simulink model "Nonlinear_PolePlacement"  (R2019b)
settings: Solver=VariableStepAuto  StartTime=0.0  StopTime=10.0  RelTol=1e-3
values from neighbouring files (symbols this model uses):
  b = 0.2    [HOMEWORK..m]
  g = 9.81    [HOMEWORK..m]
  Ktest = place(A,B,p)    [HOMEWORK..m]
  M = M_1*1.05+m    (= 11.3)    [HOMEWORK..m]
  m = 1.64    [HOMEWORK..m]
  Nu = NxNu(5)    [HOMEWORK..m]
  Nx = NxNu(1:4,:)    [HOMEWORK..m]
  x_0_1 = -0.01    [HOMEWORK..m]
  x_0_2 = 0.01    [HOMEWORK..m]
  x_0_3 = 0.05    [HOMEWORK..m]
  x_0_4 = 0.1    [HOMEWORK..m]
undefined symbols (not defined in the file or in its folder): J, L
settings Model: Creator=Sina  LastModifiedBy=Harris
settings OptimizationCC: LifeSpan=inf
settings DebuggingCC: SFExecutionAtInitializationDiag=none  ArithmeticOperatorsInVariantConditions=warning
settings SFSimCC: CustomCodeUndefinedFunction=UseInterfaceOnly
settings CodeAppCC: StateflowObjectComments=on

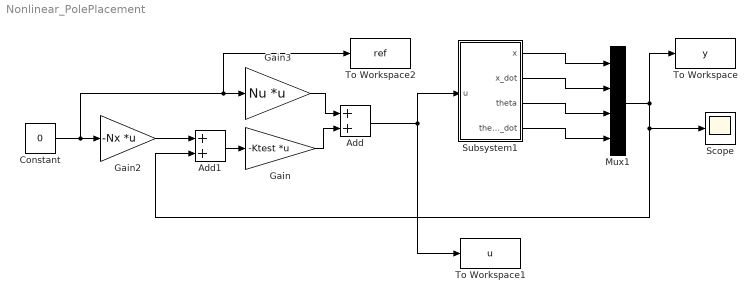
== system Nonlinear_PolePlacement ==
  Add : Sum
  Add1 : Sum
  Constant : Constant  Value=0
  Gain : Gain  Gain=-Ktest  Multiplication=Matrix(K*u) (u vector)
  Gain2 : Gain  Gain=-Nx  Multiplication=Matrix(K*u)
  Gain3 : Gain  Gain=Nu  Multiplication=Matrix(K*u)
  Mux1 : Mux
  Scope : Scope
  Subsystem1 : Subsystem
  To Workspace : ToWorkspace  VariableName=y  SaveFormat=Structure With Time  SampleTime=-1
  To Workspace1 : ToWorkspace  VariableName=u  SaveFormat=Structure With Time  SampleTime=-1
  To Workspace2 : ToWorkspace  VariableName=ref  SaveFormat=Structure With Time  SampleTime=-1
  wires:
  Add/1 -> Subsystem1/1(u), To Workspace1/1
  Constant/1 -> Gain2/1, To Workspace2/1, Gain3/1
  Gain/1 -> Add/2
  Gain2/1 -> Add1/1
  Add1/1 -> Gain/1
  Mux1/1 -> To Workspace/1, Add1/2, Scope/1
  Subsystem1/1(x) -> Mux1/1
  Subsystem1/2(x_dot) -> Mux1/2
  Subsystem1/3(theta) -> Mux1/3
  Subsystem1/4(theta_dot) -> Mux1/4
  Gain3/1 -> Add/1

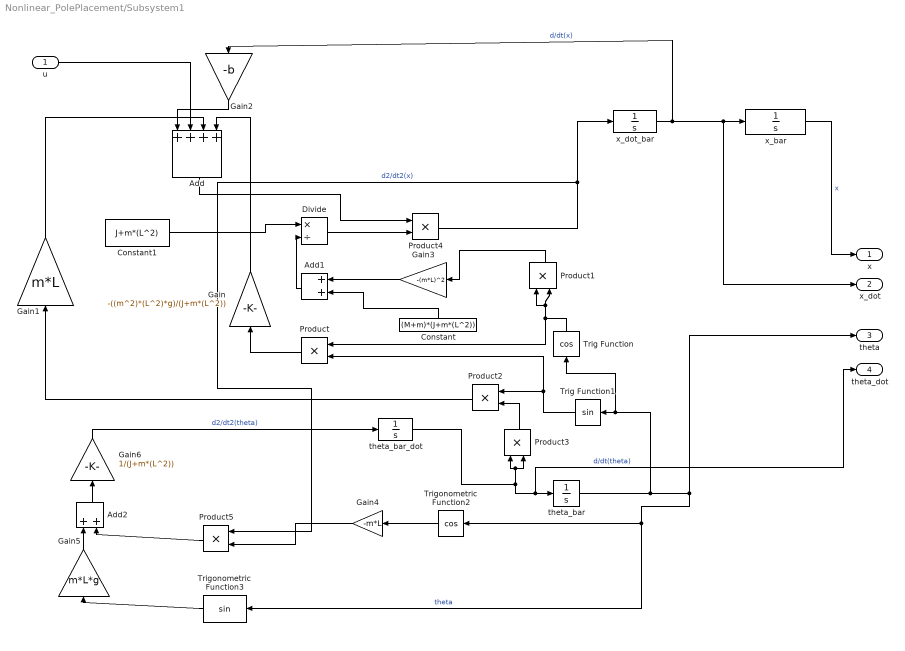
== system Nonlinear_PolePlacement/Subsystem1 ==
  u : Inport
  Add : Sum  Inputs=++++
  Add1 : Sum
  Add2 : Sum
  Constant : Constant  Value=(M+m)*(J+m*(L^2))
  Constant1 : Constant  Value=J+m*(L^2)
  Divide : Product  Inputs=*/
  Gain : Gain  Gain=-((m^2)*(L^2)*g)/(J+m*(L^2))
  Gain1 : Gain  Gain=m*L
  Gain2 : Gain  Gain=-b
  Gain3 : Gain  Gain=-(m*L)^2
  Gain4 : Gain  Gain=-m*L
  Gain5 : Gain  Gain=m*L*g
  Gain6 : Gain  Gain=1/(J+m*(L^2))
  Product{,1..5} (6 alike) : Product
  Trig Function : Trigonometry  Operator=cos
  Trig Function1 : Trigonometry
  Trigonometric Function2 : Trigonometry  Operator=cos
  Trigonometric Function3 : Trigonometry
  theta_bar : Integrator  InitialCondition=x_0_3
  theta_bar_dot : Integrator  InitialCondition=x_0_4
  x_bar : Integrator  InitialCondition=x_0_1
  x_dot_bar : Integrator  InitialCondition=x_0_2
  x : Outport
  x_dot : Outport  Port=2
  theta : Outport  Port=3
  theta_dot : Outport  Port=4
  wires:
  x_dot_bar/1 -> x_dot/1, x_bar/1, Gain2/1  "d/dt(x)"
  Trig Function/1 -> Product/1, Product1/1, Product1/2
  Product4/1 -> x_dot_bar/1, Product5/1  "d2/dt2(x)"
  x_bar/1 -> x/1  "x"
  theta_bar_dot/1 -> theta_dot/1, theta_bar/1, Product3/1, Product3/2  "d/dt(theta)"
  theta_bar/1 -> theta/1, Trigonometric Function3/1, Trigonometric Function2/1, Trig Function/1, Trig Function1/1  "theta"
  Constant/1 -> Add1/2
  Trig Function1/1 -> Product/2, Product2/1
  Product5/1 -> Add2/2
  Product3/1 -> Product2/2
  Trigonometric Function2/1 -> Gain4/1
  Gain1/1 -> Add/3
  Product2/1 -> Gain1/1
  Product/1 -> Gain/1
  Gain2/1 -> Add/1
  Gain5/1 -> Add2/1
  Trigonometric Function3/1 -> Gain5/1
  Add1/1 -> Divide/2
  Gain4/1 -> Product5/2
  Add/1 -> Product4/1
  Divide/1 -> Product4/2
  Gain6/1 -> theta_bar_dot/1  "d2/dt2(theta)"
  Add2/1 -> Gain6/1
  Gain/1 -> Add/4
  Constant1/1 -> Divide/1
  u/1 -> Add/2
  Gain3/1 -> Add1/1
  Product1/1 -> Gain3/1
